simulink model "FBL_ON_UAV_Final"  (R2024b)
settings: Solver=ode45  StartTime=0.0  StopTime=12  MaxStep=0.001  RelTol=1e-3
undefined symbols (not defined in the file or in its folder): A_inv
libraries: slpidlib x8, rllib x1, simulink x1
settings Model: Creator=shree  LastModifiedBy=shree
settings SolverCC: MaxConsecutiveMinStep=5

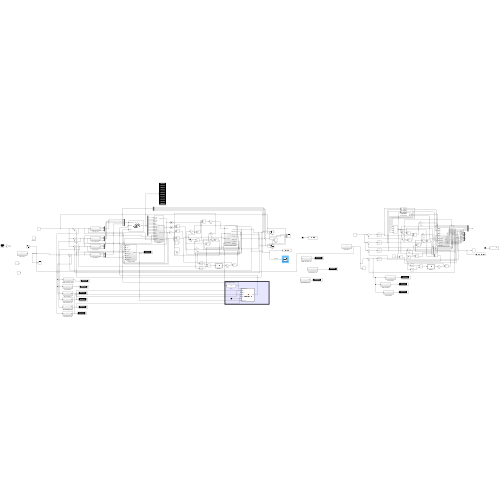
[thumbnail: Simulink's stored preview of the top-level diagram]
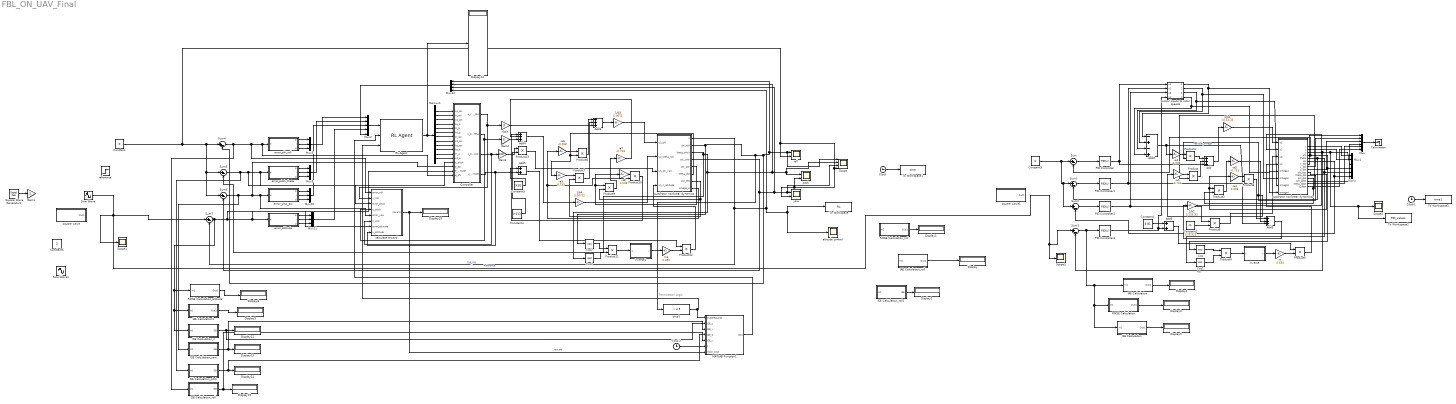
== system FBL_ON_UAV_Final ==
  note: Termination Logic
  -a1 : Gain  Gain=0.733
  -a2 : Gain  Gain=-0.008
  -a3 : Gain  Gain=-0.733
  -a4 : Gain  Gain=0.008
  -a5 : Gain  Gain=0.733
  -a6 : Gain  Gain=-0.008
  -a7 : Gain  Gain=-0.733
  -a8 : Gain  Gain=0.008
  1/b1 : Gain  Gain=1/133.33
  1/b2 : Gain  Gain=1/133.33
  1/b3 : Gain  Gain=0.0075
  1/b4 : Gain  Gain=0.00752
  Add{,1,3..4} (4 alike) : Sum  Inputs=+++
  Add2 : Sum  Inputs=-+-+
  Add5 : Sum
  Add6 : Sum
  Clock : Clock
      settings: Decimation=4
  Clock1 : Clock
  Clock2 : Clock
  Constant : Constant  Value=0
  Constant1 : Constant  Value=9.81
  Constant2 : Constant  Value=1/76.923
  Constant3 : Constant  Value=9.81
  Constant4 : Constant  Value=0.013
  Constant5 : Constant  Value=0
  Constant6 : Constant  Value=3
  Controller : Subsystem
  Cos{,1..3} (4 alike) : Trigonometry  Operator=cos
  Demux1 : Demux  Outputs=12
  Display{,1..5,8..15} (14 alike) : Display
  Gain : Gain  Gain=3
  Gain1 : Gain  Gain=-1
  Gain2 : Gain  Gain=5
  Gain3 : Gain  Gain=100
  IAE Calculation : Subsystem
  IAE Calculation1 : Subsystem
  IAE Calculation_roll : Subsystem
  ISE Calculation : Subsystem
  ISE Calculation_pitch : Subsystem
  ISE Calculation_roll : Subsystem
  ISE Calculation_roll1 : Subsystem
  ISE Calculation_yaw : Subsystem
  ISE Calculation_z : Subsystem
  MATLAB Function1 : MATLAB Function  TreatAsAtomicUnit=on  SystemSampleTime=0.1
  Mux : Mux  Inputs=6
  Mux{1,3..4,9..11} (6 alike) : Mux  Inputs=3
  Mux12 : Mux
  Mux2 : Mux  Inputs=5
  PID Controller : slpidlib/PID Controller  Controller=PID  Form=Parallel  TimeDomain=Continuous-time  UseExternalTs=off  SampleTime=-1  IntegratorMethod=Forward Euler  FilterMethod=Forward Euler  ControllerParametersSource=internal  P=50  I=50  UseKiTs=off  D=50  UseExternalDerivativeSource=off  N=200  UseFilter=on  TunerSelectOption=Transfer Function Based (PID Tuner App)  InitialConditionSource=internal  InitialConditionForIntegrator=0  InitialConditionForFilter=0  DifferentiatorICPrevScaledInput=0  ExternalReset=none  TrackingMode=off  Kt=1  LimitOutput=off  SatLimitsSource=internal  UpperSaturationLimit=inf  LowerSaturationLimit=-inf  LinearizeAsGain=on  AntiWindupMode=none  Kb=1  LimitIntegrator=off  UpperIntegratorSaturationLimit=inf  LowerIntegratorSaturationLimit=-inf  POutMin=[]  POutMax=[]  IOutMin=[]  IOutMax=[]  DOutMin=[]  DOutMax=[]  NOutMin=[]  NOutMax=[]  SumOutMin=[]  SumOutMax=[]  SaturationOutMin=[]  SaturationOutMax=[]  PParamMin=[]  PParamMax=[]  IParamMin=[]  IParamMax=[]  DParamMin=[]  DParamMax=[]  NParamMin=[]  NParamMax=[]  KbParamMin=[]  KbParamMax=[]  KtParamMin=[]  KtParamMax=[]  KbOutMin=[]  KbOutMax=[]  KtOutMin=[]  KtOutMax=[]  IntegratorOutMin=[]  IntegratorOutMax=[]  FilterOutMin=[]  FilterOutMax=[]  SumI1OutMin=[]  SumI1OutMax=[]  SumI2OutMin=[]  SumI2OutMax=[]  SumI3OutMin=[]  SumI3OutMax=[]  SumI4OutMin=[]  SumI4OutMax=[]  SumDOutMin=[]  SumDOutMax=[]  DifferentiatorOutMin=[]  DifferentiatorOutMax=[]  FilterDiffOutCoefMin=[]  FilterDiffOutCoefMax=[]  ReciprocalOutMin=[]  ReciprocalOutMax=[]  SumDenOutMin=[]  SumDenOutMax=[]  SumNumOutMin=[]  SumNumOutMax=[]  DivideOutMin=[]  DivideOutMax=[]  UdiffTsProdOutMin=[]  UdiffTsProdOutMax=[]  NTsProdOutMin=[]  NTsProdOutMax=[]  UintegralTsProdOutMin=[]  UintegralTsProdOutMax=[]  UngainTsProdOutMin=[]  UngainTsProdOutMax=[]  ClampingZeroOutDataTypeStr=Inherit: Inherit via back propagation  ClampingZeroOutMin=[]  ClampingZeroOutMax=[]  FilterDenConstantOutDataTypeStr=Inherit: Inherit via back propagation  FilterDenConstantOutMin=[]  FilterDenConstantOutMax=[]  PCopyOutDataTypeStr=Inherit: Inherit via back propagation  PCopyOutMin=[]  PCopyOutMax=[]  NCopyOutDataTypeStr=Inherit: Inherit via back propagation  NCopyOutMin=[]  NCopyOutMax=[]  IntegratorContinuousStateAttributes=''  IntegratorStateMustResolveToSignalObject=off  IntegratorRTWStateStorageClass=Auto  FilterContinuousStateAttributes=''  FilterStateMustResolveToSignalObject=off  FilterRTWStateStorageClass=Auto  ParallelPVariant=InternalParameters  IdealPVariant=Disabled  IVariant=InternalParameters  DVariant=InternalParameters  IntegratorVariant=Continuous  SatVariant=Disabled  AWVariant=Passthrough  PCopyVariant=Disabled  TRVariant=Disabled  FdbkBlocksVariant=Forward  IdealPFdbkVariant=Disabled  SatFdbkVariant=Disabled  DerivativeFilterVariant=ContFilter  NVariant=InternalParameters  NCopyVariant=Disabled  FilterICVariant=InternalICsFilter  IntegratorICVariant=InternalICs  ExternalResetVariant=Disabled  TRSumVariant=Passthrough  SumFdbkVariant=Disabled  SumVariant=Sum_PID  TsampFilterVariant=InternalTs  TsampNgainVariant=Passthrough  TsampIntegralVariant=Disabled_SignalSpec  ExternalSaturationOutDataTypeStr=Inherit: Same as second input  DerivativeSourceVariant=ErrorSignal  PreIntVariant=InternalPreInt
  PID Controller1 : slpidlib/PID Controller  Controller=PID  Form=Parallel  TimeDomain=Continuous-time  UseExternalTs=off  SampleTime=-1  IntegratorMethod=Forward Euler  FilterMethod=Forward Euler  ControllerParametersSource=internal  P=10  I=0.5  UseKiTs=off  D=10  UseExternalDerivativeSource=off  N=100  UseFilter=on  TunerSelectOption=Transfer Function Based (PID Tuner App)  InitialConditionSource=internal  InitialConditionForIntegrator=0  InitialConditionForFilter=0  DifferentiatorICPrevScaledInput=0  ExternalReset=none  TrackingMode=off  Kt=1  LimitOutput=off  SatLimitsSource=internal  UpperSaturationLimit=inf  LowerSaturationLimit=-inf  LinearizeAsGain=on  AntiWindupMode=none  Kb=1  LimitIntegrator=off  UpperIntegratorSaturationLimit=inf  LowerIntegratorSaturationLimit=-inf  POutMin=[]  POutMax=[]  IOutMin=[]  IOutMax=[]  DOutMin=[]  DOutMax=[]  NOutMin=[]  NOutMax=[]  SumOutMin=[]  SumOutMax=[]  SaturationOutMin=[]  SaturationOutMax=[]  PParamMin=[]  PParamMax=[]  IParamMin=[]  IParamMax=[]  DParamMin=[]  DParamMax=[]  NParamMin=[]  NParamMax=[]  KbParamMin=[]  KbParamMax=[]  KtParamMin=[]  KtParamMax=[]  KbOutMin=[]  KbOutMax=[]  KtOutMin=[]  KtOutMax=[]  IntegratorOutMin=[]  IntegratorOutMax=[]  FilterOutMin=[]  FilterOutMax=[]  SumI1OutMin=[]  SumI1OutMax=[]  SumI2OutMin=[]  SumI2OutMax=[]  SumI3OutMin=[]  SumI3OutMax=[]  SumI4OutMin=[]  SumI4OutMax=[]  SumDOutMin=[]  SumDOutMax=[]  DifferentiatorOutMin=[]  DifferentiatorOutMax=[]  FilterDiffOutCoefMin=[]  FilterDiffOutCoefMax=[]  ReciprocalOutMin=[]  ReciprocalOutMax=[]  SumDenOutMin=[]  SumDenOutMax=[]  SumNumOutMin=[]  SumNumOutMax=[]  DivideOutMin=[]  DivideOutMax=[]  UdiffTsProdOutMin=[]  UdiffTsProdOutMax=[]  NTsProdOutMin=[]  NTsProdOutMax=[]  UintegralTsProdOutMin=[]  UintegralTsProdOutMax=[]  UngainTsProdOutMin=[]  UngainTsProdOutMax=[]  ClampingZeroOutDataTypeStr=Inherit: Inherit via back propagation  ClampingZeroOutMin=[]  ClampingZeroOutMax=[]  FilterDenConstantOutDataTypeStr=Inherit: Inherit via back propagation  FilterDenConstantOutMin=[]  FilterDenConstantOutMax=[]  PCopyOutDataTypeStr=Inherit: Inherit via back propagation  PCopyOutMin=[]  PCopyOutMax=[]  NCopyOutDataTypeStr=Inherit: Inherit via back propagation  NCopyOutMin=[]  NCopyOutMax=[]  IntegratorContinuousStateAttributes=''  IntegratorStateMustResolveToSignalObject=off  IntegratorRTWStateStorageClass=Auto  FilterContinuousStateAttributes=''  FilterStateMustResolveToSignalObject=off  FilterRTWStateStorageClass=Auto  ParallelPVariant=InternalParameters  IdealPVariant=Disabled  IVariant=InternalParameters  DVariant=InternalParameters  IntegratorVariant=Continuous  SatVariant=Disabled  AWVariant=Passthrough  PCopyVariant=Disabled  TRVariant=Disabled  FdbkBlocksVariant=Forward  IdealPFdbkVariant=Disabled  SatFdbkVariant=Disabled  DerivativeFilterVariant=ContFilter  NVariant=InternalParameters  NCopyVariant=Disabled  FilterICVariant=InternalICsFilter  IntegratorICVariant=InternalICs  ExternalResetVariant=Disabled  TRSumVariant=Passthrough  SumFdbkVariant=Disabled  SumVariant=Sum_PID  TsampFilterVariant=InternalTs  TsampNgainVariant=Passthrough  TsampIntegralVariant=Disabled_SignalSpec  ExternalSaturationOutDataTypeStr=Inherit: Same as second input  DerivativeSourceVariant=ErrorSignal  PreIntVariant=InternalPreInt
  PID Controller2 : slpidlib/PID Controller  Controller=PID  Form=Parallel  TimeDomain=Continuous-time  UseExternalTs=off  SampleTime=-1  IntegratorMethod=Forward Euler  FilterMethod=Forward Euler  ControllerParametersSource=internal  P=43.  I=4  UseKiTs=off  D=130  UseExternalDerivativeSource=off  N=9  UseFilter=on  TunerSelectOption=Transfer Function Based (PID Tuner App)  InitialConditionSource=internal  InitialConditionForIntegrator=0  InitialConditionForFilter=0  DifferentiatorICPrevScaledInput=0  ExternalReset=none  TrackingMode=off  Kt=1  LimitOutput=off  SatLimitsSource=internal  UpperSaturationLimit=inf  LowerSaturationLimit=-inf  LinearizeAsGain=on  AntiWindupMode=none  Kb=1  LimitIntegrator=off  UpperIntegratorSaturationLimit=inf  LowerIntegratorSaturationLimit=-inf  POutMin=[]  POutMax=[]  IOutMin=[]  IOutMax=[]  DOutMin=[]  DOutMax=[]  NOutMin=[]  NOutMax=[]  SumOutMin=[]  SumOutMax=[]  SaturationOutMin=[]  SaturationOutMax=[]  PParamMin=[]  PParamMax=[]  IParamMin=[]  IParamMax=[]  DParamMin=[]  DParamMax=[]  NParamMin=[]  NParamMax=[]  KbParamMin=[]  KbParamMax=[]  KtParamMin=[]  KtParamMax=[]  KbOutMin=[]  KbOutMax=[]  KtOutMin=[]  KtOutMax=[]  IntegratorOutMin=[]  IntegratorOutMax=[]  FilterOutMin=[]  FilterOutMax=[]  SumI1OutMin=[]  SumI1OutMax=[]  SumI2OutMin=[]  SumI2OutMax=[]  SumI3OutMin=[]  SumI3OutMax=[]  SumI4OutMin=[]  SumI4OutMax=[]  SumDOutMin=[]  SumDOutMax=[]  DifferentiatorOutMin=[]  DifferentiatorOutMax=[]  FilterDiffOutCoefMin=[]  FilterDiffOutCoefMax=[]  ReciprocalOutMin=[]  ReciprocalOutMax=[]  SumDenOutMin=[]  SumDenOutMax=[]  SumNumOutMin=[]  SumNumOutMax=[]  DivideOutMin=[]  DivideOutMax=[]  UdiffTsProdOutMin=[]  UdiffTsProdOutMax=[]  NTsProdOutMin=[]  NTsProdOutMax=[]  UintegralTsProdOutMin=[]  UintegralTsProdOutMax=[]  UngainTsProdOutMin=[]  UngainTsProdOutMax=[]  ClampingZeroOutDataTypeStr=Inherit: Inherit via back propagation  ClampingZeroOutMin=[]  ClampingZeroOutMax=[]  FilterDenConstantOutDataTypeStr=Inherit: Inherit via back propagation  FilterDenConstantOutMin=[]  FilterDenConstantOutMax=[]  PCopyOutDataTypeStr=Inherit: Inherit via back propagation  PCopyOutMin=[]  PCopyOutMax=[]  NCopyOutDataTypeStr=Inherit: Inherit via back propagation  NCopyOutMin=[]  NCopyOutMax=[]  IntegratorContinuousStateAttributes=''  IntegratorStateMustResolveToSignalObject=off  IntegratorRTWStateStorageClass=Auto  FilterContinuousStateAttributes=''  FilterStateMustResolveToSignalObject=off  FilterRTWStateStorageClass=Auto  ParallelPVariant=InternalParameters  IdealPVariant=Disabled  IVariant=InternalParameters  DVariant=InternalParameters  IntegratorVariant=Continuous  SatVariant=Disabled  AWVariant=Passthrough  PCopyVariant=Disabled  TRVariant=Disabled  FdbkBlocksVariant=Forward  IdealPFdbkVariant=Disabled  SatFdbkVariant=Disabled  DerivativeFilterVariant=ContFilter  NVariant=InternalParameters  NCopyVariant=Disabled  FilterICVariant=InternalICsFilter  IntegratorICVariant=InternalICs  ExternalResetVariant=Disabled  TRSumVariant=Passthrough  SumFdbkVariant=Disabled  SumVariant=Sum_PID  TsampFilterVariant=InternalTs  TsampNgainVariant=Passthrough  TsampIntegralVariant=Disabled_SignalSpec  ExternalSaturationOutDataTypeStr=Inherit: Same as second input  DerivativeSourceVariant=ErrorSignal  PreIntVariant=InternalPreInt
  PID Controller3 : slpidlib/PID Controller  Controller=PID  Form=Parallel  TimeDomain=Continuous-time  UseExternalTs=off  SampleTime=-1  IntegratorMethod=Forward Euler  FilterMethod=Forward Euler  ControllerParametersSource=internal  P=100  I=10  UseKiTs=off  D=100  UseExternalDerivativeSource=off  N=100  UseFilter=on  TunerSelectOption=Transfer Function Based (PID Tuner App)  InitialConditionSource=internal  InitialConditionForIntegrator=0  InitialConditionForFilter=0  DifferentiatorICPrevScaledInput=0  ExternalReset=none  TrackingMode=off  Kt=1  LimitOutput=off  SatLimitsSource=internal  UpperSaturationLimit=inf  LowerSaturationLimit=-inf  LinearizeAsGain=on  AntiWindupMode=none  Kb=1  LimitIntegrator=off  UpperIntegratorSaturationLimit=inf  LowerIntegratorSaturationLimit=-inf  POutMin=[]  POutMax=[]  IOutMin=[]  IOutMax=[]  DOutMin=[]  DOutMax=[]  NOutMin=[]  NOutMax=[]  SumOutMin=[]  SumOutMax=[]  SaturationOutMin=[]  SaturationOutMax=[]  PParamMin=[]  PParamMax=[]  IParamMin=[]  IParamMax=[]  DParamMin=[]  DParamMax=[]  NParamMin=[]  NParamMax=[]  KbParamMin=[]  KbParamMax=[]  KtParamMin=[]  KtParamMax=[]  KbOutMin=[]  KbOutMax=[]  KtOutMin=[]  KtOutMax=[]  IntegratorOutMin=[]  IntegratorOutMax=[]  FilterOutMin=[]  FilterOutMax=[]  SumI1OutMin=[]  SumI1OutMax=[]  SumI2OutMin=[]  SumI2OutMax=[]  SumI3OutMin=[]  SumI3OutMax=[]  SumI4OutMin=[]  SumI4OutMax=[]  SumDOutMin=[]  SumDOutMax=[]  DifferentiatorOutMin=[]  DifferentiatorOutMax=[]  FilterDiffOutCoefMin=[]  FilterDiffOutCoefMax=[]  ReciprocalOutMin=[]  ReciprocalOutMax=[]  SumDenOutMin=[]  SumDenOutMax=[]  SumNumOutMin=[]  SumNumOutMax=[]  DivideOutMin=[]  DivideOutMax=[]  UdiffTsProdOutMin=[]  UdiffTsProdOutMax=[]  NTsProdOutMin=[]  NTsProdOutMax=[]  UintegralTsProdOutMin=[]  UintegralTsProdOutMax=[]  UngainTsProdOutMin=[]  UngainTsProdOutMax=[]  ClampingZeroOutDataTypeStr=Inherit: Inherit via back propagation  ClampingZeroOutMin=[]  ClampingZeroOutMax=[]  FilterDenConstantOutDataTypeStr=Inherit: Inherit via back propagation  FilterDenConstantOutMin=[]  FilterDenConstantOutMax=[]  PCopyOutDataTypeStr=Inherit: Inherit via back propagation  PCopyOutMin=[]  PCopyOutMax=[]  NCopyOutDataTypeStr=Inherit: Inherit via back propagation  NCopyOutMin=[]  NCopyOutMax=[]  IntegratorContinuousStateAttributes=''  IntegratorStateMustResolveToSignalObject=off  IntegratorRTWStateStorageClass=Auto  FilterContinuousStateAttributes=''  FilterStateMustResolveToSignalObject=off  FilterRTWStateStorageClass=Auto  ParallelPVariant=InternalParameters  IdealPVariant=Disabled  IVariant=InternalParameters  DVariant=InternalParameters  IntegratorVariant=Continuous  SatVariant=Disabled  AWVariant=Passthrough  PCopyVariant=Disabled  TRVariant=Disabled  FdbkBlocksVariant=Forward  IdealPFdbkVariant=Disabled  SatFdbkVariant=Disabled  DerivativeFilterVariant=ContFilter  NVariant=InternalParameters  NCopyVariant=Disabled  FilterICVariant=InternalICsFilter  IntegratorICVariant=InternalICs  ExternalResetVariant=Disabled  TRSumVariant=Passthrough  SumFdbkVariant=Disabled  SumVariant=Sum_PID  TsampFilterVariant=InternalTs  TsampNgainVariant=Passthrough  TsampIntegralVariant=Disabled_SignalSpec  ExternalSaturationOutDataTypeStr=Inherit: Same as second input  DerivativeSourceVariant=ErrorSignal  PreIntVariant=InternalPreInt
  Product{,1..13} (14 alike) : Product
  RL Agent : rllib/RL Agent  Agent=agent_TD3_Final  ExternalActionAsInput=off  ProvideLastAction=off  ProvideCumRwd=off  TreatAsDirectFeedthrough=on  UseStrictObservationDataTypes=off
  RMSE Calculation : Subsystem
  RMSE Calculation_altitude : Subsystem
  RMSE Calculation_roll : Subsystem
  Scope : Scope  NumInputPorts=4
  Scope1 : Scope
  Scope2 : Scope
  Scope3 : Scope
  Sine Wave : Sin  Amplitude=3  Frequency=3  SampleTime=0
  Sine Wave1 : Sin  Amplitude=3  SampleTime=0
  Square Wave Generator1 : SignalGenerator  WaveForm=square  Amplitude=3
  Sum{,1..7} (8 alike) : Sum  Inputs=|+-
  Terminator : Terminator
  To Workspace : ToWorkspace  VariableName=RL  SaveFormat=Timeseries  SampleTime=-1
  To Workspace1 : ToWorkspace  VariableName=time  SaveFormat=Timeseries  SampleTime=-1
  To Workspace2 : ToWorkspace  VariableName=PID_values  SaveFormat=Structure With Time  SampleTime=-1
  To Workspace3 : ToWorkspace  VariableName=time1  SaveFormat=Timeseries  SampleTime=-1
  altitude control : Scope
  calculate reward : Subsystem
  cmp1 : simulink/Logic and Bit Operations/Compare To Constant  relop=>  const=3.5  OutDataTypeStr=boolean
  control inputs to rotor speeds : Subsystem
  error_altitude : Subsystem
  error_phi_roll : Subsystem
  error_pitch_theta : Subsystem
  error_yaw_psi : Subsystem
  inverse : MATLAB Function  TreatAsAtomicUnit=on
  inverse1 : MATLAB Function  TreatAsAtomicUnit=on
  m : Gain  Gain=0.650
  m1 : Gain  Gain=0.650
  pitch : Scope  NumInputPorts=2
  quadrotor nonlinear dynamics : Subsystem
  quadrotor nonlinear dynamics1 : Subsystem
  reference : Step  Time=0  After=3  SampleTime=0.1
  roll : Scope  NumInputPorts=2
  square wave : Subsystem
  square wave1 : Subsystem
  yaw : Scope  NumInputPorts=2
  wires:
  Demux1/9 -> Controller/9(kp_psi)
  Mux11/1 -> Mux2/4
  Product7/1 -> Add1/2
  Sum7/1 -> ISE Calculation_z/1(In1), IAE Calculation1/1(In1), RMSE Calculation_altitude/1(In1), Controller/15(e_altitude), calculate reward/7(error_altitude), error_altitude/1(e)
  RMSE Calculation_altitude/1(Out1) -> Display8/1
  Demux1/3 -> Controller/3(kd_phi)
  Product9/1 -> -a7/1
  quadrotor nonlinear dynamics/7(psi_dot) -> Product9/2, Product7/2
  -a6/1 -> Product8/1
  quadrotor nonlinear dynamics/5(phi_dot) -> -a8/1, Product9/1
  Demux1/5 -> Controller/5(ki_p)
  error_pitch_theta/1(p) -> Mux9/1
  error_phi_roll/3(d) -> Mux3/3
  Cos3/1 -> Product11/2
  calculate reward/1(reward) -> MATLAB Function1/7(input_cost), Display10/1  "reward"
  Mux2/1 -> RL Agent/1
  error_altitude/3(d) -> Mux11/3
  Product10/1 -> Add4/1
  Demux1/1 -> Controller/1(kp_phi)
  Clock2/1 -> MATLAB Function1/6(t)
  Mux3/1 -> Mux2/1
  error_phi_roll/1(p) -> Mux3/1
  RL Agent/1 -> Display12/1, Demux1/1
  -a7/1 -> Add4/2
  Demux1/6 -> Controller/6(kd_p)
  quadrotor nonlinear dynamics/4(psi_yaw) -> Sum6/2, Scope/3, yaw/1, Mux12/3
  Mux10/1 -> Mux2/3
  error_altitude/1(p) -> Mux11/1
  Controller/3(u_psi_yaw) -> Gain3/1, calculate reward/6(u_yaw)
  ISE Calculation_pitch/1(ISE) -> MATLAB Function1/4(ISE_p), Display14/1
  Product12/1 -> quadrotor nonlinear dynamics/4(u4_z_altitude)
  Controller/1(u_roll_phii) -> calculate reward/2(u_roll), Gain/1
  Sum5/1 -> ISE Calculation_pitch/1(In1), calculate reward/3(error_pitch), Controller/13(e_pitch), error_pitch_theta/1(e)
  Sum4/1 -> ISE Calculation_roll/1(In1), calculate reward/1(error_roll), Controller/16(e_phi), error_phi_roll/1(e)
  Mux9/1 -> Mux2/2
  error_pitch_theta/2(i) -> Mux9/2
  Controller/2(u_pitch_theta) -> calculate reward/4(u_pitch), Gain2/1
  Constant3/1 -> Add5/1
  ISE Calculation_z/1(ISE) -> MATLAB Function1/2(ISE_z), Display11/1
  cmp1/1 -> MATLAB Function1/1(OutOfBounds), RL Agent/3
  m1/1 -> Product12/2
  error_phi_roll/2(i) -> Mux3/2
  error_altitude/2(i) -> Mux11/2
  Demux1/12 -> Controller/12(kd_a)
  -a8/1 -> Product10/1
  error_yaw_psi/3(d) -> Mux10/3
  quadrotor nonlinear dynamics/1(z) -> Sum7/2, altitude control/1, To Workspace/1, Mux12/4  "TD3_PID"
  Demux1/10 -> Controller/10(kp_a)
  Demux1/4 -> Controller/4(kp_p)
  error_yaw_psi/1(p) -> Mux10/1
  MATLAB Function1/1(cost) -> RL Agent/2
  error_yaw_psi/2(i) -> Mux10/2
  Cos2/1 -> Product11/1
  Add4/1 -> 1/b4/1
  Sum6/1 -> ISE Calculation_yaw/1(In1), Controller/14(e_psi), calculate reward/5(error_yaw), error_yaw_psi/1(e)
  Demux1/11 -> Controller/11(ki_a)
  Product11/1 -> inverse1/1(u)
  Demux1/2 -> Controller/2(ki_phi)
  Add1/1 -> 1/b3/1
  ISE Calculation_yaw/1(ISE) -> MATLAB Function1/3(ISE_y), Display13/1
  Product8/1 -> Add1/1
  Add5/1 -> Product12/1
  Demux1/7 -> Controller/7(ki_psi)
  Constant4/1 -> Product13/2
  -a5/1 -> Product7/1
  inverse1/1(y) -> m1/1
  Demux1/8 -> Controller/8(kd_psi)
  1/b4/1 -> quadrotor nonlinear dynamics/2(u2_theta_roll)
  quadrotor nonlinear dynamics/6(theta_dot) -> -a5/1, Product8/2
  ISE Calculation_roll/1(ISE) -> MATLAB Function1/5(ISE_r), Display15/1
  quadrotor nonlinear dynamics/2(phi_roll) -> cmp1/1, Sum4/2, Mux12/1, Scope/1, roll/1, Cos2/1
  Square Wave Generator1/1 -> Gain1/1
  IAE Calculation1/1(Out1) -> Display9/1
  error_pitch_theta/3(d) -> Mux9/3
  Product13/1 -> quadrotor nonlinear dynamics/3(u3_psi_yaw)
  Mux12/1 -> Mux2/5
  quadrotor nonlinear dynamics/8(omega_d) -> Product10/2, -a6/1
  Sine Wave/1 -> Sum3/1, Scope3/1, Scope1/1, Sum7/1  "Reference"
  Gain/1 -> Add1/3
  Gain2/1 -> Add4/3
  Gain3/1 -> Product13/1
  Controller/4(u_altitude) -> Add5/2, calculate reward/8(u_altitude)
  IAE Calculation_roll/1(Out1) -> Display/1
  RMSE Calculation_roll/1(Out1) -> Display1/1
  ISE Calculation_roll1/1(ISE) -> Display2/1
  1/b3/1 -> quadrotor nonlinear dynamics/1(u1_phi)
  quadrotor nonlinear dynamics/3(theta_pitch) -> Sum5/2, Mux12/2, Scope/2, pitch/1, Cos3/1
  Clock/1 -> To Workspace1/1
  Constant/1 -> roll/2, yaw/2, pitch/2, Scope/4, Sum6/1, Sum5/1, Sum4/1
  Mux/1 -> Terminator/1
  quadrotor nonlinear dynamics1/3(z) -> Sum3/2, To Workspace2/1, Scope2/1, Mux1/3  "PID"
  RMSE Calculation/1(Out1) -> Display3/1
  quadrotor nonlinear dynamics1/9(z_dot) -> Mux/3
  control inputs to rotor speeds/4(omega4) -> quadrotor nonlinear dynamics1/8(omega4), Add2/4
  Product2/1 -> -a3/1
  quadrotor nonlinear dynamics1/10(phi_dot) -> -a4/1, Product2/1
  quadrotor nonlinear dynamics1/7(x_dot) -> Mux/1
  Constant1/1 -> Add6/1
  Constant2/1 -> Product6/2
  Sum1/1 -> PID Controller1/1
  control inputs to rotor speeds/3(omega3) -> quadrotor nonlinear dynamics1/7(omega3), Add2/3
  Product4/1 -> inverse/1(u)
  quadrotor nonlinear dynamics1/13(phi_ddot) -> Mux/4
  -a2/1 -> Product1/1
  Product1/1 -> Add/1
  quadrotor nonlinear dynamics1/6(psi) -> Sum2/2, Mux4/3
  Sum/1 -> PID Controller/1
  quadrotor nonlinear dynamics1/15(z_ddot) -> Mux/6
  Cos1/1 -> Product4/2
  quadrotor nonlinear dynamics1/12(psi_dot) -> Product2/2, Product/2
  Sum3/1 -> ISE Calculation/1(In1), RMSE Calculation/1(In1), IAE Calculation/1(In1), PID Controller3/1
  control inputs to rotor speeds/2(omega2) -> quadrotor nonlinear dynamics1/6(omega2), Add2/2
  Add/1 -> 1/b1/1
  -a1/1 -> Product/1
  m/1 -> Product5/2
  quadrotor nonlinear dynamics1/2(y) -> Mux1/2
  quadrotor nonlinear dynamics1/5(theta) -> Sum1/2, Mux4/2, Cos1/1
  quadrotor nonlinear dynamics1/8(y_dot) -> Mux/2
  ISE Calculation/1(Out1) -> Display5/1
  control inputs to rotor speeds/1(omega1) -> quadrotor nonlinear dynamics1/5(omega1), Add2/1
  1/b2/1 -> quadrotor nonlinear dynamics1/2(u2)
  Product5/1 -> quadrotor nonlinear dynamics1/4(u4)
  Product3/1 -> Add3/1
  quadrotor nonlinear dynamics1/4(phi) -> Sum/2, Cos/1, Mux4/1
  Constant5/1 -> Sum2/1, Sum1/1, Sum/1
  Product/1 -> Add/2
  -a3/1 -> Add3/2
  quadrotor nonlinear dynamics1/11(theta_dot) -> Product1/2, -a1/1
  PID Controller1/1 -> control inputs to rotor speeds/2(u2), Add3/3
  PID Controller/1 -> Add/3, control inputs to rotor speeds/1(u1)
  Add3/1 -> 1/b2/1
  1/b1/1 -> quadrotor nonlinear dynamics1/1(u1)
  Sum2/1 -> PID Controller2/1
  Add6/1 -> Product5/1
  PID Controller2/1 -> control inputs to rotor speeds/3(u3), Product6/1
  Clock1/1 -> To Workspace3/1
  IAE Calculation/1(Out1) -> Display4/1
  -a4/1 -> Product3/1
  PID Controller3/1 -> control inputs to rotor speeds/4(u4), Add6/2
  quadrotor nonlinear dynamics1/14(theta_ddot) -> Mux/5
  Cos/1 -> Product4/1
  Product6/1 -> quadrotor nonlinear dynamics1/3(u3)
  inverse/1(y) -> m/1
  Add2/1 -> -a2/1, Product3/2  "residual_omega"
  quadrotor nonlinear dynamics1/1(x) -> Mux1/1

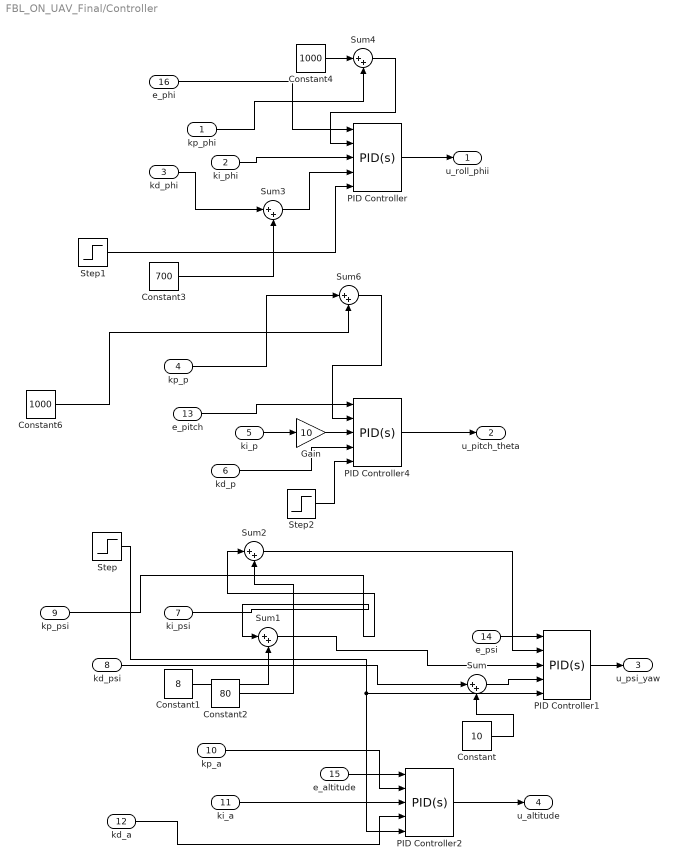
== system FBL_ON_UAV_Final/Controller ==
  kp_phi : Inport
  ki_phi : Inport  Port=2
  kd_phi : Inport  Port=3
  kp_p : Inport  Port=4
  ki_p : Inport  Port=5
  kd_p : Inport  Port=6
  ki_psi : Inport  Port=7
  kd_psi : Inport  Port=8
  kp_psi : Inport  Port=9
  kp_a : Inport  Port=10
  ki_a : Inport  Port=11
  kd_a : Inport  Port=12
  e_pitch : Inport  Port=13
  e_psi : Inport  Port=14
  e_altitude : Inport  Port=15
  e_phi : Inport  Port=16
  Constant : Constant  Value=10
  Constant1 : Constant  Value=8
  Constant2 : Constant  Value=80
  Constant3 : Constant  Value=700
  Constant4 : Constant  Value=1000
  Constant6 : Constant  Value=1000
  Gain : Gain  Gain=10
  PID Controller{,1..2,4} (4 alike) : slpidlib/PID Controller  Controller=PID  Form=Parallel  TimeDomain=Continuous-time  UseExternalTs=off  SampleTime=0.1  IntegratorMethod=Forward Euler  FilterMethod=Forward Euler  ControllerParametersSource=external  P=1  I=1  UseKiTs=off  D=0  UseExternalDerivativeSource=off  N=100  UseFilter=on  TunerSelectOption=Transfer Function Based (PID Tuner App)  InitialConditionSource=internal  InitialConditionForIntegrator=0  InitialConditionForFilter=0  DifferentiatorICPrevScaledInput=0  ExternalReset=none  TrackingMode=off  Kt=1  LimitOutput=off  SatLimitsSource=internal  UpperSaturationLimit=inf  LowerSaturationLimit=-inf  LinearizeAsGain=on  AntiWindupMode=none  Kb=1  LimitIntegrator=off  UpperIntegratorSaturationLimit=inf  LowerIntegratorSaturationLimit=-inf  POutMin=[]  POutMax=[]  IOutMin=[]  IOutMax=[]  DOutMin=[]  DOutMax=[]  NOutMin=[]  NOutMax=[]  SumOutMin=[]  SumOutMax=[]  SaturationOutMin=[]  SaturationOutMax=[]  PParamMin=[]  PParamMax=[]  IParamMin=[]  IParamMax=[]  DParamMin=[]  DParamMax=[]  NParamMin=[]  NParamMax=[]  KbParamMin=[]  KbParamMax=[]  KtParamMin=[]  KtParamMax=[]  KbOutMin=[]  KbOutMax=[]  KtOutMin=[]  KtOutMax=[]  IntegratorOutMin=[]  IntegratorOutMax=[]  FilterOutMin=[]  FilterOutMax=[]  SumI1OutMin=[]  SumI1OutMax=[]  SumI2OutMin=[]  SumI2OutMax=[]  SumI3OutMin=[]  SumI3OutMax=[]  SumI4OutMin=[]  SumI4OutMax=[]  SumDOutMin=[]  SumDOutMax=[]  DifferentiatorOutMin=[]  DifferentiatorOutMax=[]  FilterDiffOutCoefMin=[]  FilterDiffOutCoefMax=[]  ReciprocalOutMin=[]  ReciprocalOutMax=[]  SumDenOutMin=[]  SumDenOutMax=[]  SumNumOutMin=[]  SumNumOutMax=[]  DivideOutMin=[]  DivideOutMax=[]  UdiffTsProdOutMin=[]  UdiffTsProdOutMax=[]  NTsProdOutMin=[]  NTsProdOutMax=[]  UintegralTsProdOutMin=[]  UintegralTsProdOutMax=[]  UngainTsProdOutMin=[]  UngainTsProdOutMax=[]  ClampingZeroOutDataTypeStr=Inherit: Inherit via back propagation  ClampingZeroOutMin=[]  ClampingZeroOutMax=[]  FilterDenConstantOutDataTypeStr=Inherit: Inherit via back propagation  FilterDenConstantOutMin=[]  FilterDenConstantOutMax=[]  PCopyOutDataTypeStr=Inherit: Inherit via back propagation  PCopyOutMin=[]  PCopyOutMax=[]  NCopyOutDataTypeStr=Inherit: Inherit via back propagation  NCopyOutMin=[]  NCopyOutMax=[]  IntegratorContinuousStateAttributes=''  IntegratorStateMustResolveToSignalObject=off  IntegratorRTWStateStorageClass=Auto  FilterContinuousStateAttributes=''  FilterStateMustResolveToSignalObject=off  FilterRTWStateStorageClass=Auto  ParallelPVariant=ExternalParameters  IdealPVariant=Disabled  IVariant=ExternalParameters  DVariant=ExternalParameters  IntegratorVariant=Continuous  SatVariant=Disabled  AWVariant=Passthrough  PCopyVariant=Disabled  TRVariant=Disabled  FdbkBlocksVariant=Forward  IdealPFdbkVariant=Disabled  SatFdbkVariant=Disabled  DerivativeFilterVariant=ContFilter  NVariant=ExternalParameters  NCopyVariant=Disabled  FilterICVariant=InternalICsFilter  IntegratorICVariant=InternalICs  ExternalResetVariant=Disabled  TRSumVariant=Passthrough  SumFdbkVariant=Disabled  SumVariant=Sum_PID  TsampFilterVariant=InternalTs  TsampNgainVariant=Passthrough  TsampIntegralVariant=Disabled_SignalSpec  ExternalSaturationOutDataTypeStr=Inherit: Same as second input  DerivativeSourceVariant=ErrorSignal  PreIntVariant=InternalPreInt
  Step : Step  Time=0  After=800  SampleTime=0.1
  Step1 : Step  Time=0  After=800  SampleTime=0.1
  Step2 : Step  Time=0  After=700  SampleTime=0.1
  Sum{,1..4,6} (6 alike) : Sum  Inputs=|++
  u_roll_phii : Outport
  u_pitch_theta : Outport  Port=2
  u_psi_yaw : Outport  Port=3
  u_altitude : Outport  Port=4
  wires:
  Step/1 -> PID Controller2/5, PID Controller1/5
  e_phi/1 -> PID Controller/1
  PID Controller/1 -> u_roll_phii/1
  PID Controller4/1 -> u_pitch_theta/1
  PID Controller2/1 -> u_altitude/1
  e_altitude/1 -> PID Controller2/1
  e_psi/1 -> PID Controller1/1
  PID Controller1/1 -> u_psi_yaw/1
  kp_a/1 -> PID Controller2/2
  ki_a/1 -> PID Controller2/3
  kd_a/1 -> PID Controller2/4
  kp_psi/1 -> Sum2/1
  ki_psi/1 -> Sum1/1
  kd_psi/1 -> Sum/1
  Constant/1 -> Sum/2
  Sum/1 -> PID Controller1/4
  Constant1/1 -> Sum1/2
  Sum1/1 -> PID Controller1/3
  Sum2/1 -> PID Controller1/2
  Constant2/1 -> Sum2/2
  kp_phi/1 -> Sum4/2
  kd_phi/1 -> Sum3/1
  e_pitch/1 -> PID Controller4/1
  ki_p/1 -> Gain/1
  Step1/1 -> PID Controller/5
  Step2/1 -> PID Controller4/5
  kp_p/1 -> Sum6/1
  kd_p/1 -> PID Controller4/4
  Gain/1 -> PID Controller4/3
  Sum3/1 -> PID Controller/4
  Constant4/1 -> Sum4/1
  Sum4/1 -> PID Controller/2
  ki_phi/1 -> PID Controller/3
  Constant6/1 -> Sum6/2
  Sum6/1 -> PID Controller4/2
  Constant3/1 -> Sum3/2

== system FBL_ON_UAV_Final/IAE Calculation ==
  In1 : Inport
  Abs : Abs  SaturateOnIntegerOverflow=off
  Integrator6 : Integrator
  Out1 : Outport
  wires:
  Abs/1 -> Integrator6/1
  Integrator6/1 -> Out1/1
  In1/1 -> Abs/1

== system FBL_ON_UAV_Final/IAE Calculation1 ==
  In1 : Inport
  Abs : Abs  SaturateOnIntegerOverflow=off
  Integrator6 : Integrator
  Out1 : Outport
  wires:
  Abs/1 -> Integrator6/1
  Integrator6/1 -> Out1/1
  In1/1 -> Abs/1

== system FBL_ON_UAV_Final/IAE Calculation_roll ==
  In1 : Inport
  Abs : Abs  SaturateOnIntegerOverflow=off
  Integrator6 : Integrator
  Out1 : Outport
  wires:
  Abs/1 -> Integrator6/1
  Integrator6/1 -> Out1/1
  In1/1 -> Abs/1

== system FBL_ON_UAV_Final/ISE Calculation ==
  In1 : Inport
  Integrator6 : Integrator
  Square : Math  Operator=square
  Out1 : Outport
  wires:
  Square/1 -> Integrator6/1
  Integrator6/1 -> Out1/1
  In1/1 -> Square/1

== system FBL_ON_UAV_Final/ISE Calculation_pitch ==
  In1 : Inport
  Integrator6 : Integrator
  Square : Math  Operator=square
  ISE : Outport
  wires:
  Square/1 -> Integrator6/1
  Integrator6/1 -> ISE/1
  In1/1 -> Square/1

== system FBL_ON_UAV_Final/ISE Calculation_roll ==
  In1 : Inport
  Integrator6 : Integrator
  Square : Math  Operator=square
  ISE : Outport
  wires:
  Square/1 -> Integrator6/1
  Integrator6/1 -> ISE/1
  In1/1 -> Square/1

== system FBL_ON_UAV_Final/ISE Calculation_roll1 ==
  In1 : Inport
  Integrator6 : Integrator
  Square : Math  Operator=square
  ISE : Outport
  wires:
  Square/1 -> Integrator6/1
  Integrator6/1 -> ISE/1
  In1/1 -> Square/1

== system FBL_ON_UAV_Final/ISE Calculation_yaw ==
  In1 : Inport
  Integrator6 : Integrator
  Square : Math  Operator=square
  ISE : Outport
  wires:
  Square/1 -> Integrator6/1
  Integrator6/1 -> ISE/1
  In1/1 -> Square/1

== system FBL_ON_UAV_Final/ISE Calculation_z ==
  In1 : Inport
  Integrator6 : Integrator
  Square : Math  Operator=square
  ISE : Outport
  wires:
  Square/1 -> Integrator6/1
  Integrator6/1 -> ISE/1
  In1/1 -> Square/1

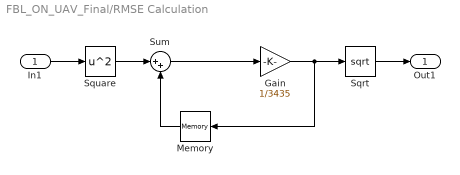
== system FBL_ON_UAV_Final/RMSE Calculation ==
  In1 : Inport
  Gain : Gain  Gain=1/3435
  Memory : Memory
  Sqrt : Sqrt
  Square : Math  Operator=square
  Sum : Sum  Inputs=|++
  Out1 : Outport
  wires:
  In1/1 -> Square/1
  Square/1 -> Sum/1
  Memory/1 -> Sum/2
  Sum/1 -> Gain/1
  Gain/1 -> Sqrt/1, Memory/1
  Sqrt/1 -> Out1/1

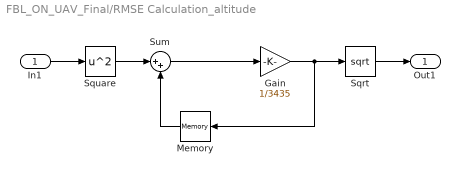
== system FBL_ON_UAV_Final/RMSE Calculation_altitude ==
  In1 : Inport
  Gain : Gain  Gain=1/3435
  Memory : Memory
  Sqrt : Sqrt
  Square : Math  Operator=square
  Sum : Sum  Inputs=|++
  Out1 : Outport
  wires:
  In1/1 -> Square/1
  Square/1 -> Sum/1
  Memory/1 -> Sum/2
  Sum/1 -> Gain/1
  Gain/1 -> Sqrt/1, Memory/1
  Sqrt/1 -> Out1/1

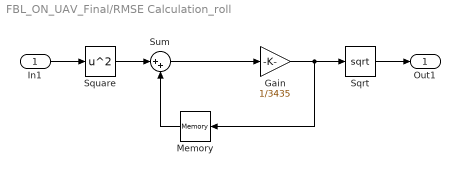
== system FBL_ON_UAV_Final/RMSE Calculation_roll ==
  In1 : Inport
  Gain : Gain  Gain=1/3435
  Memory : Memory
  Sqrt : Sqrt
  Square : Math  Operator=square
  Sum : Sum  Inputs=|++
  Out1 : Outport
  wires:
  In1/1 -> Square/1
  Square/1 -> Sum/1
  Memory/1 -> Sum/2
  Sum/1 -> Gain/1
  Gain/1 -> Sqrt/1, Memory/1
  Sqrt/1 -> Out1/1

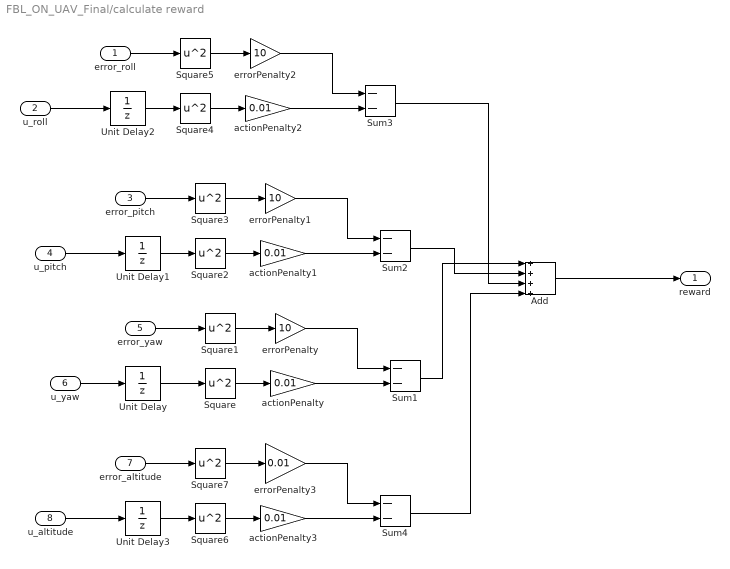
== system FBL_ON_UAV_Final/calculate reward ==
  error_roll : Inport
  u_roll : Inport  Port=2
  error_pitch : Inport  Port=3
  u_pitch : Inport  Port=4
  error_yaw : Inport  Port=5
  u_yaw : Inport  Port=6
  error_altitude : Inport  Port=7
  u_altitude : Inport  Port=8
  Add : Sum  Inputs=++++
  Square{,1..7} (8 alike) : Math  Operator=square
  Sum{1..4} (4 alike) : Sum  Inputs=--  OutDataTypeStr=double
  Unit Delay{,1..3} (4 alike) : UnitDelay  SampleTime=-1  HasFrameUpgradeWarning=on
  actionPenalty{,1..3} (4 alike) : Gain  Gain=0.01
  errorPenalty : Gain  Gain=10
  errorPenalty1 : Gain  Gain=10
  errorPenalty2 : Gain  Gain=10
  errorPenalty3 : Gain  Gain=0.01
  reward : Outport
  wires:
  Square1/1 -> errorPenalty/1
  errorPenalty/1 -> Sum1/1
  actionPenalty/1 -> Sum1/2
  Square/1 -> actionPenalty/1
  u_yaw/1 -> Unit Delay/1
  error_yaw/1 -> Square1/1
  Sum1/1 -> Add/1
  Square3/1 -> errorPenalty1/1
  Square2/1 -> actionPenalty1/1
  error_pitch/1 -> Square3/1
  u_pitch/1 -> Unit Delay1/1
  errorPenalty1/1 -> Sum2/1
  Sum2/1 -> Add/2
  actionPenalty1/1 -> Sum2/2
  Square5/1 -> errorPenalty2/1
  Square4/1 -> actionPenalty2/1
  error_roll/1 -> Square5/1
  u_roll/1 -> Unit Delay2/1
  errorPenalty2/1 -> Sum3/1
  Sum3/1 -> Add/3
  actionPenalty2/1 -> Sum3/2
  Square7/1 -> errorPenalty3/1
  Square6/1 -> actionPenalty3/1
  error_altitude/1 -> Square7/1
  u_altitude/1 -> Unit Delay3/1
  errorPenalty3/1 -> Sum4/1
  Sum4/1 -> Add/4
  actionPenalty3/1 -> Sum4/2
  Unit Delay/1 -> Square/1
  Unit Delay1/1 -> Square2/1
  Unit Delay2/1 -> Square4/1
  Unit Delay3/1 -> Square6/1
  Add/1 -> reward/1

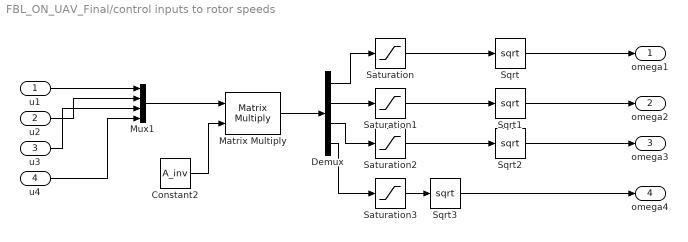
== system FBL_ON_UAV_Final/control inputs to rotor speeds ==
  u1 : Inport
  u2 : Inport  Port=2
  u3 : Inport  Port=3
  u4 : Inport  Port=4
  Constant2 : Constant  Value=A_inv
  Demux : Demux
  Matrix Multiply : Product  Multiplication=Matrix(*)
  Mux1 : Mux
  Saturation{,1..3} (4 alike) : Saturate  UpperLimit=360000  LowerLimit=0
  Sqrt{,1..3} (4 alike) : Sqrt
  omega1 : Outport
  omega2 : Outport  Port=2
  omega3 : Outport  Port=3
  omega4 : Outport  Port=4
  wires:
  Demux/1 -> Saturation/1
  u1/1 -> Mux1/1
  Demux/2 -> Saturation1/1
  u2/1 -> Mux1/2
  Saturation3/1 -> Sqrt3/1
  Saturation2/1 -> Sqrt2/1
  Saturation/1 -> Sqrt/1
  Matrix Multiply/1 -> Demux/1
  Mux1/1 -> Matrix Multiply/1
  u4/1 -> Mux1/4
  Constant2/1 -> Matrix Multiply/2
  Saturation1/1 -> Sqrt1/1
  Demux/3 -> Saturation2/1
  Demux/4 -> Saturation3/1
  Sqrt2/1 -> omega3/1
  Sqrt/1 -> omega1/1
  u3/1 -> Mux1/3
  Sqrt3/1 -> omega4/1
  Sqrt1/1 -> omega2/1

== system FBL_ON_UAV_Final/error_altitude ==
  e : Inport
  Derivative : Derivative
  Integrator : Integrator
  p : Outport
  i : Outport  Port=2
  d : Outport  Port=3
  wires:
  Integrator/1 -> i/1
  e/1 -> Derivative/1, Integrator/1, p/1
  Derivative/1 -> d/1

== system FBL_ON_UAV_Final/error_phi_roll ==
  e : Inport
  Derivative : Derivative
  Integrator : Integrator
  p : Outport
  i : Outport  Port=2
  d : Outport  Port=3
  wires:
  Integrator/1 -> i/1
  e/1 -> p/1, Derivative/1, Integrator/1
  Derivative/1 -> d/1

== system FBL_ON_UAV_Final/error_pitch_theta ==
  e : Inport
  Derivative : Derivative
  Integrator : Integrator
  p : Outport
  i : Outport  Port=2
  d : Outport  Port=3
  wires:
  Integrator/1 -> i/1
  e/1 -> p/1, Derivative/1, Integrator/1
  Derivative/1 -> d/1

== system FBL_ON_UAV_Final/error_yaw_psi ==
  e : Inport
  Derivative : Derivative
  Integrator : Integrator
  p : Outport
  i : Outport  Port=2
  d : Outport  Port=3
  wires:
  Integrator/1 -> i/1
  e/1 -> p/1, Derivative/1, Integrator/1
  Derivative/1 -> d/1

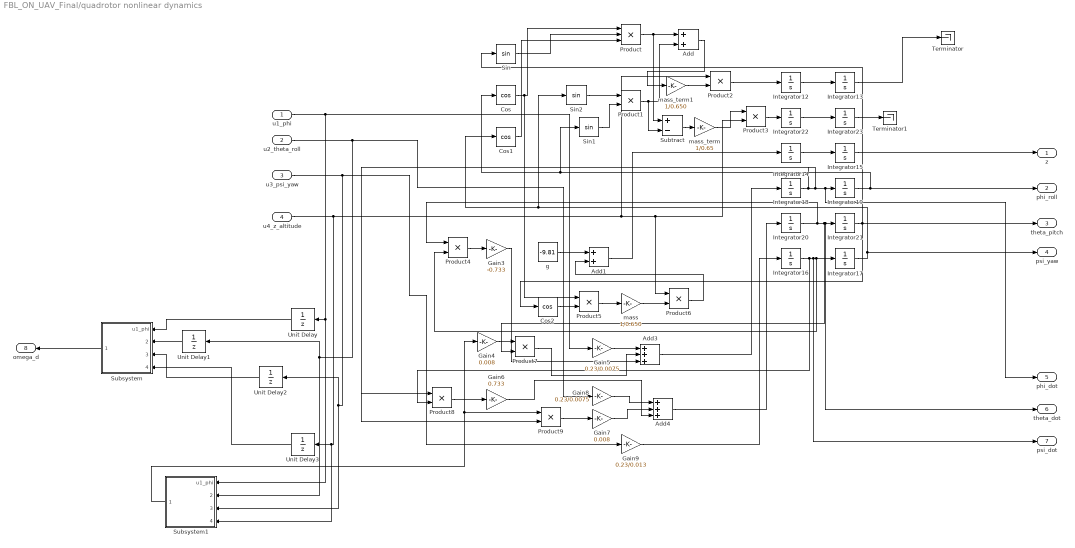
== system FBL_ON_UAV_Final/quadrotor nonlinear dynamics ==
  u1_phi : Inport
  u2_theta_roll : Inport  Port=2
  u3_psi_yaw : Inport  Port=3
  u4_z_altitude : Inport  Port=4
  Add : Sum
  Add1 : Sum
  Add3 : Sum  Inputs=+++
  Add4 : Sum  Inputs=+++
  Cos : Trigonometry  Operator=cos
  Cos1 : Trigonometry  Operator=cos
  Cos2 : Trigonometry  Operator=cos
  Gain3 : Gain  Gain=-0.733
  Gain4 : Gain  Gain=0.008
  Gain5 : Gain  Gain=0.23/0.0075
  Gain6 : Gain  Gain=0.733
  Gain7 : Gain  Gain=0.008
  Gain8 : Gain  Gain=0.23/0.0075
  Gain9 : Gain  Gain=0.23/0.013
  Integrator{12..15,18,20,22..23} (8 alike) : Integrator
  Integrator16 : Integrator  LowerSaturationLimit=0
  Integrator17 : Integrator  InitialCondition=1  LowerSaturationLimit=0
  Integrator19 : Integrator  InitialCondition=1  LowerSaturationLimit=0
  Integrator21 : Integrator  InitialCondition=1  LowerSaturationLimit=0
  Product : Product  Inputs=3
  Product{1..9} (9 alike) : Product
  Sin : Trigonometry
  Sin1 : Trigonometry
  Sin2 : Trigonometry
  Subsystem : Subsystem
  Subsystem1 : Subsystem
  Subtract : Sum  Inputs=+-
  Terminator : Terminator
  Terminator1 : Terminator
  Unit Delay{,1..3} (4 alike) : UnitDelay  SampleTime=-1  HasFrameUpgradeWarning=on
  g : Constant  Value=-9.81
  mass : Gain  Gain=1/0.650
  mass_term : Gain  Gain=1/0.65
  mass_term1 : Gain  Gain=1/0.650
  z : Outport
  phi_roll : Outport  Port=2
  theta_pitch : Outport  Port=3
  psi_yaw : Outport  Port=4
  phi_dot : Outport  Port=5
  theta_dot : Outport  Port=6
  psi_dot : Outport  Port=7
  omega_d : Outport  Port=8
  wires:
  Gain9/1 -> Integrator16/1
  Product9/1 -> Gain7/1
  Gain6/1 -> Add4/3
  Add3/1 -> Integrator18/1
  Add4/1 -> Integrator20/1
  Gain7/1 -> Add4/2
  Gain4/1 -> Product7/1
  Product7/1 -> Add3/2
  Product1/1 -> Subtract/2, Add/2
  g/1 -> Add1/1
  mass_term/1 -> Product3/1
  Integrator18/1 -> Product9/2, Product8/1, phi_dot/1, Integrator19/1
  mass/1 -> Product6/2
  Gain8/1 -> Add4/1
  mass_term1/1 -> Product2/2
  Gain5/1 -> Add3/1
  Product5/1 -> mass/1
  Integrator12/1 -> Integrator13/1
  Product/1 -> Subtract/1, Add/1
  Product2/1 -> Integrator12/1
  Integrator15/1 -> z/1
  Integrator22/1 -> Integrator23/1
  Add1/1 -> Integrator14/1
  Integrator14/1 -> Integrator15/1
  Cos1/1 -> Product/3
  Cos/1 -> Product5/1, Product/1
  Integrator17/1 -> Sin2/1, Cos1/1, psi_yaw/1
  Sin1/1 -> Product1/2
  Integrator20/1 -> theta_dot/1, Integrator21/1, Product7/2, Product4/1
  Integrator16/1 -> Product8/2, Product4/2, Integrator17/1, psi_dot/1
  Integrator21/1 -> theta_pitch/1, Cos2/1, Sin/1
  Add/1 -> mass_term1/1
  Product4/1 -> Gain3/1
  Product6/1 -> Add1/2
  Sin2/1 -> Product1/1
  Product8/1 -> Gain6/1
  Sin/1 -> Product/2
  Cos2/1 -> Product5/2
  Product3/1 -> Integrator22/1
  Subtract/1 -> mass_term/1
  Gain3/1 -> Add3/3
  Integrator19/1 -> Sin1/1, Cos/1, phi_roll/1
  u1_phi/1 -> Subsystem1/1(u1_phi), Unit Delay/1, Gain5/1
  u4_z_altitude/1 -> Product3/2, Product6/1, Product2/1, Subsystem1/4(u4_z_altitude), Unit Delay3/1
  u3_psi_yaw/1 -> Subsystem1/3(u3_psi_yaw), Unit Delay2/1, Gain9/1
  u2_theta_roll/1 -> Subsystem1/2(u2_theta_roll), Unit Delay1/1, Gain8/1
  Unit Delay/1 -> Subsystem/1(u1_phi)
  Unit Delay1/1 -> Subsystem/2(u2_theta_roll)
  Unit Delay2/1 -> Subsystem/3(u3_psi_yaw)
  Unit Delay3/1 -> Subsystem/4(u4_z_altitude)
  Integrator13/1 -> Terminator/1
  Integrator23/1 -> Terminator1/1
  Subsystem/1(omega_d) -> omega_d/1
  Subsystem1/1(omega_d) -> Product9/1, Gain4/1

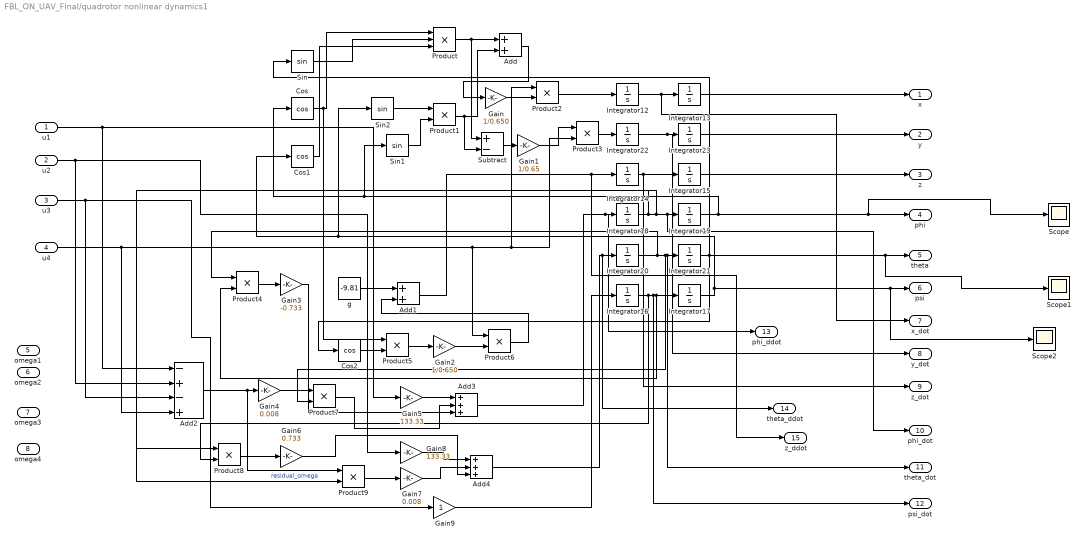
== system FBL_ON_UAV_Final/quadrotor nonlinear dynamics1 ==
  u1 : Inport
  u2 : Inport  Port=2
  u3 : Inport  Port=3
  u4 : Inport  Port=4
  omega1 : Inport  Port=5
  omega2 : Inport  Port=6
  omega3 : Inport  Port=7
  omega4 : Inport  Port=8
  Add : Sum
  Add1 : Sum
  Add2 : Sum  Inputs=-+-+
  Add3 : Sum  Inputs=+++
  Add4 : Sum  Inputs=+++
  Cos : Trigonometry  Operator=cos
  Cos1 : Trigonometry  Operator=cos
  Cos2 : Trigonometry  Operator=cos
  Gain : Gain  Gain=1/0.650
  Gain1 : Gain  Gain=1/0.65
  Gain2 : Gain  Gain=1/0.650
  Gain3 : Gain  Gain=-0.733
  Gain4 : Gain  Gain=0.008
  Gain5 : Gain  Gain=133.33
  Gain6 : Gain  Gain=0.733
  Gain7 : Gain  Gain=0.008
  Gain8 : Gain  Gain=133.33
  Gain9 : Gain
  Integrator{12..16,18,20,22..23} (9 alike) : Integrator
  Integrator17 : Integrator  InitialCondition=1  LowerSaturationLimit=0
  Integrator19 : Integrator  InitialCondition=1  LowerSaturationLimit=0
  Integrator21 : Integrator  InitialCondition=1  LowerSaturationLimit=0
  Product : Product  Inputs=3
  Product{1..9} (9 alike) : Product
  Scope : Scope
  Scope1 : Scope
  Scope2 : Scope
  Sin : Trigonometry
  Sin1 : Trigonometry
  Sin2 : Trigonometry
  Subtract : Sum  Inputs=+-
  g : Constant  Value=-9.81
  x : Outport
  y : Outport  Port=2
  z : Outport  Port=3
  phi : Outport  Port=4
  theta : Outport  Port=5
  psi : Outport  Port=6
  x_dot : Outport  Port=7
  y_dot : Outport  Port=8
  z_dot : Outport  Port=9
  phi_dot : Outport  Port=10
  theta_dot : Outport  Port=11
  psi_dot : Outport  Port=12
  phi_ddot : Outport  Port=13
  theta_ddot : Outport  Port=14
  z_ddot : Outport  Port=15
  wires:
  Gain9/1 -> Integrator16/1
  Product9/1 -> Gain7/1
  Gain6/1 -> Add4/3
  Add3/1 -> phi_ddot/1, Integrator18/1
  Add4/1 -> theta_ddot/1, Integrator20/1
  Gain7/1 -> Add4/2
  u3/1 -> Add2/3, Gain9/1
  Add2/1 -> Product9/1, Gain4/1  "residual_omega"
  Gain4/1 -> Product7/1
  u2/1 -> Add2/2, Gain8/1
  Product7/1 -> Add3/2
  Product1/1 -> Subtract/2, Add/2
  g/1 -> Add1/1
  Gain1/1 -> Product3/1
  Integrator18/1 -> Product9/2, Product8/1, phi_dot/1, Integrator19/1
  Gain2/1 -> Product6/2
  Gain8/1 -> Add4/1
  Gain/1 -> Product2/2
  Gain5/1 -> Add3/1
  Product5/1 -> Gain2/1
  Integrator12/1 -> x_dot/1, Integrator13/1
  Product/1 -> Subtract/1, Add/1
  Product2/1 -> Integrator12/1
  Integrator19/1 -> Sin1/1, Cos/1, Scope/1, phi/1
  Integrator15/1 -> z/1
  Integrator22/1 -> y_dot/1, Integrator23/1
  Add1/1 -> z_ddot/1, Integrator14/1
  Integrator14/1 -> Integrator15/1, z_dot/1
  Cos1/1 -> Product/3
  Cos/1 -> Product5/1, Product/1
  Integrator23/1 -> y/1
  Integrator17/1 -> Sin2/1, Cos1/1, Scope2/1, psi/1
  Sin1/1 -> Product1/2
  Integrator20/1 -> theta_dot/1, Integrator21/1, Product7/2, Product4/1
  Integrator16/1 -> Product8/2, Integrator17/1, Product4/2, psi_dot/1
  u4/1 -> Add2/4, Product6/1, Product3/2, Product2/1
  Integrator21/1 -> Scope1/1, theta/1, Cos2/1, Sin/1
  Add/1 -> Gain/1
  Product4/1 -> Gain3/1
  u1/1 -> Add2/1, Gain5/1
  Integrator13/1 -> x/1
  Product6/1 -> Add1/2
  Sin2/1 -> Product1/1
  Product8/1 -> Gain6/1
  Sin/1 -> Product/2
  Cos2/1 -> Product5/2
  Product3/1 -> Integrator22/1
  Subtract/1 -> Gain1/1
  Gain3/1 -> Add3/3

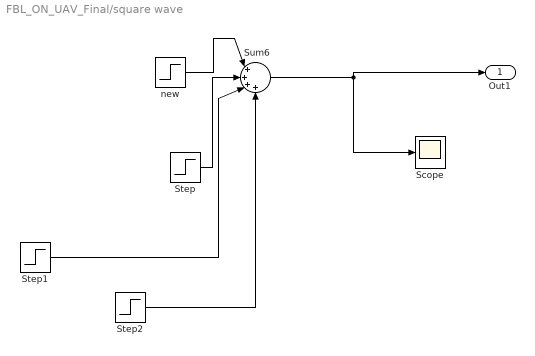
== system FBL_ON_UAV_Final/square wave ==
  Scope : Scope
  Step : Step  Time=4  SampleTime=0
  Step1 : Step  Time=8  After=-1  SampleTime=0
  Step2 : Step  Time=10  After=-1  SampleTime=0
  Sum6 : Sum  Inputs=|++++
  new : Step  Time=2  SampleTime=0.1
  Out1 : Outport
  wires:
  Sum6/1 -> Out1/1, Scope/1
  Step/1 -> Sum6/2
  new/1 -> Sum6/1
  Step1/1 -> Sum6/3
  Step2/1 -> Sum6/4

== system FBL_ON_UAV_Final/square wave1 ==
  Scope : Scope
  Step : Step  Time=4  SampleTime=0
  Step1 : Step  Time=8  After=-1  SampleTime=0
  Step2 : Step  Time=10  After=-1  SampleTime=0
  Sum6 : Sum  Inputs=|++++
  new : Step  Time=2  SampleTime=0.1
  Out1 : Outport
  wires:
  Sum6/1 -> Out1/1, Scope/1
  Step/1 -> Sum6/2
  new/1 -> Sum6/1
  Step1/1 -> Sum6/3
  Step2/1 -> Sum6/4

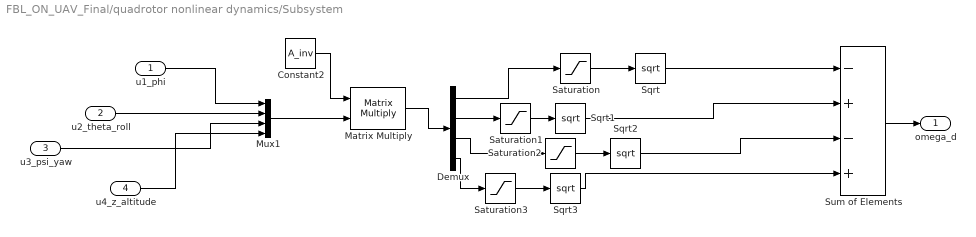
== system FBL_ON_UAV_Final/quadrotor nonlinear dynamics/Subsystem ==
  u1_phi : Inport
  u2_theta_roll : Inport  Port=2
  u3_psi_yaw : Inport  Port=3
  u4_z_altitude : Inport  Port=4
  Constant2 : Constant  Value=A_inv
  Demux : Demux
  Matrix Multiply : Product  Multiplication=Matrix(*)
  Mux1 : Mux
  Saturation{,1..3} (4 alike) : Saturate  UpperLimit=490000  LowerLimit=0
  Sqrt{,1..3} (4 alike) : Sqrt
  Sum of Elements : Sum  Inputs=-+-+
  omega_d : Outport
  wires:
  Mux1/1 -> Matrix Multiply/2
  Saturation2/1 -> Sqrt2/1
  Demux/4 -> Saturation3/1
  u1_phi/1 -> Mux1/1
  Sqrt1/1 -> Sum of Elements/2
  Sqrt/1 -> Sum of Elements/1
  Saturation1/1 -> Sqrt1/1
  Constant2/1 -> Matrix Multiply/1
  Saturation/1 -> Sqrt/1
  Matrix Multiply/1 -> Demux/1
  Saturation3/1 -> Sqrt3/1
  Demux/2 -> Saturation1/1
  Demux/1 -> Saturation/1
  Demux/3 -> Saturation2/1
  Sqrt2/1 -> Sum of Elements/3
  u3_psi_yaw/1 -> Mux1/3
  u2_theta_roll/1 -> Mux1/2
  Sqrt3/1 -> Sum of Elements/4
  u4_z_altitude/1 -> Mux1/4
  Sum of Elements/1 -> omega_d/1

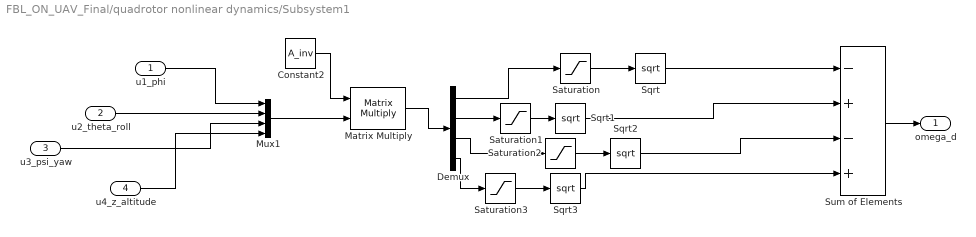
== system FBL_ON_UAV_Final/quadrotor nonlinear dynamics/Subsystem1 ==
  u1_phi : Inport
  u2_theta_roll : Inport  Port=2
  u3_psi_yaw : Inport  Port=3
  u4_z_altitude : Inport  Port=4
  Constant2 : Constant  Value=A_inv
  Demux : Demux
  Matrix Multiply : Product  Multiplication=Matrix(*)
  Mux1 : Mux
  Saturation{,1..3} (4 alike) : Saturate  UpperLimit=490000  LowerLimit=0
  Sqrt{,1..3} (4 alike) : Sqrt
  Sum of Elements : Sum  Inputs=-+-+
  omega_d : Outport
  wires:
  Mux1/1 -> Matrix Multiply/2
  Saturation2/1 -> Sqrt2/1
  Demux/4 -> Saturation3/1
  u1_phi/1 -> Mux1/1
  Sqrt1/1 -> Sum of Elements/2
  Sqrt/1 -> Sum of Elements/1
  Saturation1/1 -> Sqrt1/1
  Constant2/1 -> Matrix Multiply/1
  Saturation/1 -> Sqrt/1
  Matrix Multiply/1 -> Demux/1
  Saturation3/1 -> Sqrt3/1
  Demux/2 -> Saturation1/1
  Demux/1 -> Saturation/1
  Demux/3 -> Saturation2/1
  Sqrt2/1 -> Sum of Elements/3
  u3_psi_yaw/1 -> Mux1/3
  u2_theta_roll/1 -> Mux1/2
  Sqrt3/1 -> Sum of Elements/4
  u4_z_altitude/1 -> Mux1/4
  Sum of Elements/1 -> omega_d/1

== matlab function FBL_ON_UAV_Final/inverse ==
  data: u input; y output
function y = fcn(u)

y = 1/u;

== matlab function FBL_ON_UAV_Final/MATLAB Function1 ==
  data: OutOfBounds input; cost output; ISE_z input; ISE_y input; ISE_p input; ISE_r input; t input; input_cost input
function cost = stoppingCriterion(OutOfBounds, ISE_z, ISE_y, ISE_p, ISE_r, t, input_cost)
simEndTime = 10;
epsilon = 0.05;

if OutOfBounds
    cost = input_cost-100;
elseif (t >= simEndTime - epsilon) && (ISE_z < 0.2) && (ISE_p < 0.2) && (ISE_y < 0.2) && (ISE_r < 0.2)
    cost = input_cost+10;
else
    cost = input_cost;
end

== matlab function FBL_ON_UAV_Final/inverse1 ==
  data: u input; y output
function y = fcn(u)

y = 1/u;
